simulink library "ESTS_TFY_FLatTir"  (R2023b)
settings: Solver=VariableStepAuto  StartTime=0.0  StopTime=10.0  RelTol=1e-3
settings Model: Creator=blatak  LastModifiedBy=blatak
settings ModelReferenceCC: EnableRefExpFcnMdlSchedulingChecks=on

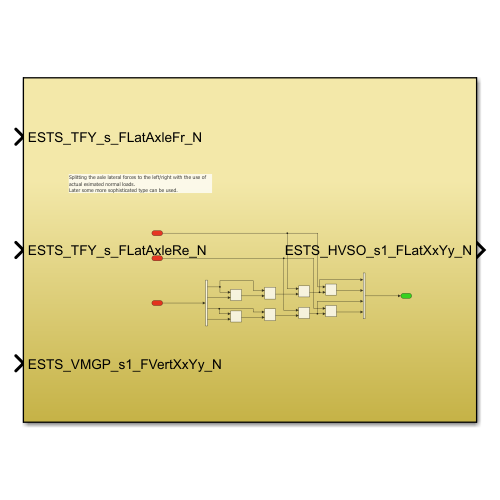
[thumbnail: Simulink's stored preview of the top-level diagram]
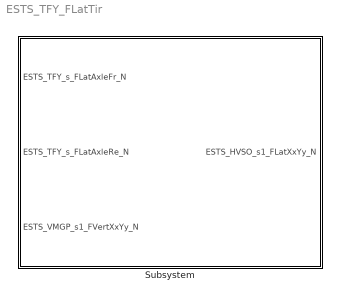
== system ESTS_TFY_FLatTir ==
  Subsystem : Subsystem

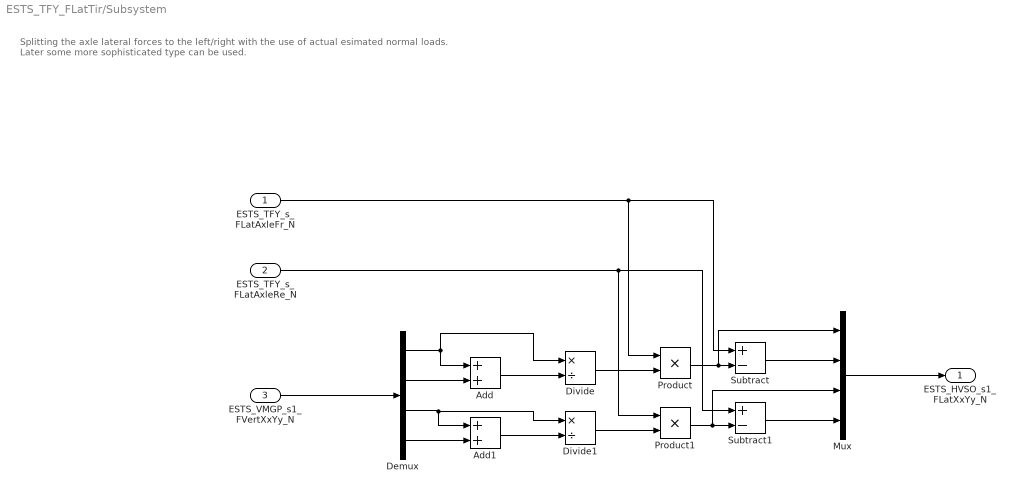
== system ESTS_TFY_FLatTir/Subsystem ==
  note: Splitting the axle lateral forces to the left/right with the use of actual esimated normal loads.
      | Later some more sophisticated type can be used.
  ESTS_TFY_s_FLatAxleFr_N : Inport
  ESTS_TFY_s_FLatAxleRe_N : Inport  Port=2
  ESTS_VMGP_s1_FVertXxYy_N : Inport  Port=3
  Add : Sum
  Add1 : Sum
  Demux : Demux
  Divide : Product  Inputs=*/  RndMeth=Zero  SaturateOnIntegerOverflow=on
  Divide1 : Product  Inputs=*/  RndMeth=Zero  SaturateOnIntegerOverflow=on
  Mux : Mux
  Product : Product
  Product1 : Product
  Subtract : Sum  Inputs=+-
  Subtract1 : Sum  Inputs=+-
  ESTS_HVSO_s1_FLatXxYy_N : Outport
  wires:
  ESTS_VMGP_s1_FVertXxYy_N/1 -> Demux/1
  Demux/1 -> Add/1, Divide/1
  Demux/2 -> Add/2
  Add/1 -> Divide/2
  Divide/1 -> Product/2
  ESTS_TFY_s_FLatAxleFr_N/1 -> Subtract/1, Product/1
  Demux/3 -> Divide1/1, Add1/1
  Demux/4 -> Add1/2
  Add1/1 -> Divide1/2
  Divide1/1 -> Product1/2
  ESTS_TFY_s_FLatAxleRe_N/1 -> Subtract1/1, Product1/1
  Product/1 -> Mux/1, Subtract/2
  Product1/1 -> Mux/3, Subtract1/2
  Subtract/1 -> Mux/2
  Subtract1/1 -> Mux/4
  Mux/1 -> ESTS_HVSO_s1_FLatXxYy_N/1
